simulink model "parte2_eje1_GeneradorSincrono"  (R2019b)
settings: Solver=VariableStepAuto  StartTime=0.0  StopTime=0.05  RelTol=1e-3
values from neighbouring files (symbols this model uses):
  id = It*sind(di+fi)    [parte2_eje1_GSin_constantes.m]
  ifd = (Et*cosd(di)+Ra*iq+Ld*id)/Lad    [parte2_eje1_GSin_constantes.m]
  iq = It*cosd(di+fi)    [parte2_eje1_GSin_constantes.m]
  L0 = 0.01    [parte2_eje1_GSin_constantes.m]
  L11d = 0.1713    [parte2_eje1_GSin_constantes.m]
  L11q = 0.7252    [parte2_eje1_GSin_constantes.m]
  L22q = 0.125    [parte2_eje1_GSin_constantes.m]
  Lad = sat*Lad    (= 1.38278)    [parte2_eje1_GSin_constantes.m]
  Laq = sat*Laq    (= 1.34113)    [parte2_eje1_GSin_constantes.m]
  Lf1d = 1.61    [parte2_eje1_GSin_constantes.m]
  Lffd = 0.165    [parte2_eje1_GSin_constantes.m]
  Ll = 0.15    [parte2_eje1_GSin_constantes.m]
  R1d = 0.0284    [parte2_eje1_GSin_constantes.m]
  R1q = 0.00619    [parte2_eje1_GSin_constantes.m]
  R2q = 0.02368    [parte2_eje1_GSin_constantes.m]
  Ra = 0.003    [parte2_eje1_GSin_constantes.m]
  Rfd = 0.0006    [parte2_eje1_GSin_constantes.m]
  th = 12*pi/180    (= 0.209439510239)    [parte2_eje1_GSin_constantes.m]
  wr = 1    [parte2_eje1_GSin_constantes.m]
settings Model: Creator=cjuar  LastModifiedBy=cjuar
settings DataIOCC: ReturnWorkspaceOutputs=off
settings DebuggingCC: ArithmeticOperatorsInVariantConditions=warning
settings SFSimCC: SimUseLocalCustomCode=off  CustomCodeUndefinedFunction=UseInterfaceOnly
settings RTWCC: RTWUseLocalCustomCode=off

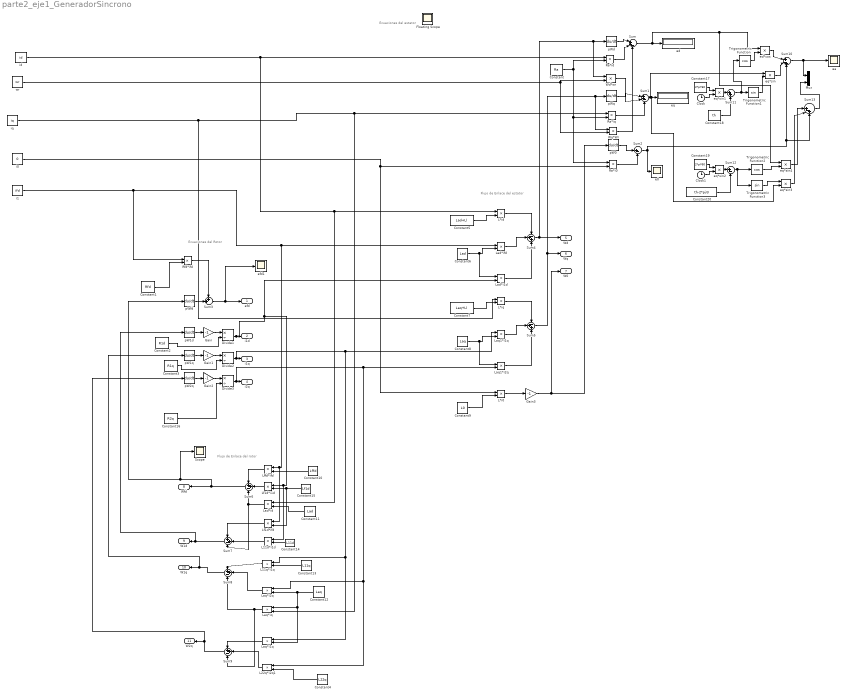
== system parte2_eje1_GeneradorSincrono ==
  note: Flujo de Enlace del estator
  note: Ecuaciones del Rotor
  note: Ecuaciones del estator
  note: Flujo de Enlace del rotor
  Clock : Clock
  Clock1 : Clock
  Constant : Constant  Value=Ra
  Constant1 : Constant  Value=Rfd
  Constant10 : Constant  Value=Lffd
  Constant11 : Constant  Value=Lad
  Constant12 : Constant  Value=Laq
  Constant13 : Constant  Value=L11q
  Constant14 : Constant  Value=L11d
  Constant15 : Constant  Value=Lf1d
  Constant16 : Constant  Value=R2q
  Constant17 : Constant  Value=2*pi*60
  Constant18 : Constant  Value=th
  Constant19 : Constant  Value=2*pi*60
  Constant2 : Constant  Value=R1d
  Constant20 : Constant  Value=th-2*pi/3
  Constant3 : Constant  Value=R1q
  Constant4 : Constant  Value=L22q
  Constant5 : Constant  Value=Lad+Ll
  Constant6 : Constant  Value=Lad
  Constant7 : Constant  Value=Laq+Ll
  Constant8 : Constant  Value=Laq
  Constant9 : Constant  Value=L0
  Divide1 : Product  Inputs=*/
  Divide2 : Product  Inputs=*/
  Divide3 : Product  Inputs=*/
  Floating Scope : Scope
      settings: Floating=on
  Gain{,1..3} (4 alike) : Gain  Gain=-1
  L*i0 : Product
  L*id : Product
  L*iq : Product
  L11d*i1d : Product
  L11q*i1q : Product
  L22q*i2q1 : Product
  Lad*i1d : Product
  Lad*id : Product
  Lad*ifd : Product
  Laq*i1q : Product
  Laq*i2q : Product
  Laq*iq : Product
  Laq1*i1q : Product
  Laq1*i2q : Product
  Lf1d*i1d : Product
  Lf1d*ifd : Product
  Lffd*ifd : Product
  Mux : Mux  Inputs=2
  Ra*i0 : Product
  Ra*id : Product
  "Ra*iq " : Product
  Rfd*ifd : Product
  Scope : Scope
  Sum : Sum  Inputs=|+--
  Sum1 : Sum  Inputs=|++-
  Sum10 : Sum  Inputs=|+-+
  Sum11 : Sum  Inputs=|++
  Sum12 : Sum  Inputs=|+-
  Sum13 : Sum  Inputs=||+-+
  Sum2 : Sum  Inputs=|+-
  Sum3 : Sum  Inputs=++|
  Sum4 : Sum  Inputs=-++
  Sum5 : Sum  Inputs=-++
  Sum{6..9} (4 alike) : Sum  Inputs=++-
  Trigonometric Function : Trigonometry  Operator=cos
  Trigonometric Function1 : Trigonometry
  Trigonometric Function2 : Trigonometry  Operator=cos
  Trigonometric Function3 : Trigonometry
  Wd*wr : Product
  Wq*Wr : Product
  e0 : Scope
  ea : Scope
  ed : Display
  ed*cos : Product
  efd1 : Scope
  eq : Display
  eq*sin{,1..4} (5 alike) : Product
  i0 : Constant  Value=0
  i1 : Constant  Value=ifd
  id : Constant  Value=id
  iq : Constant  Value=iq
  pW0 : Derivative
  pW1d : Derivative
  pW1q : Derivative
  pW2q : Derivative
  pWd : Derivative
  pWfd : Derivative
  pWq : Derivative
  wr : Constant  Value=wr
  efd : Outport  VectorParamsAs1DForOutWhenUnconnected=off
  i1d : Outport  Port=2  VectorParamsAs1DForOutWhenUnconnected=off
  i1q : Outport  Port=3  VectorParamsAs1DForOutWhenUnconnected=off
  i2q : Outport  Port=4  VectorParamsAs1DForOutWhenUnconnected=off
  Wd : Outport  Port=5  VectorParamsAs1DForOutWhenUnconnected=off
  Wq : Outport  Port=6  VectorParamsAs1DForOutWhenUnconnected=off
  W0 : Outport  Port=7  VectorParamsAs1DForOutWhenUnconnected=off
  Wfd : Outport  Port=8  VectorParamsAs1DForOutWhenUnconnected=off
  W1d : Outport  Port=9  VectorParamsAs1DForOutWhenUnconnected=off
  W1q : Outport  Port=10  VectorParamsAs1DForOutWhenUnconnected=off
  W2q : Outport  Port=11  VectorParamsAs1DForOutWhenUnconnected=off
  wires:
  Sum4/1 -> Wd/1, Wd*wr/1, pWd/1
  Sum5/1 -> Wq*Wr/1, pWq/1, Wq/1
  Gain3/1 -> W0/1, pW0/1
  wr/1 -> Wd*wr/2, Wq*Wr/2
  Sum/1 -> ed/1, eq*sin4/1, ed*cos/1
  pWd/1 -> Sum/1
  pWq/1 -> Sum1/1
  Sum1/1 -> eq*sin3/2, eq/1, eq*sin/1
  Wd*wr/1 -> Sum1/2
  Constant/1 -> Ra*id/2, Ra*i0/1, "Ra*iq "/2
  iq/1 -> "Ra*iq "/1, Laq*iq/2, L*iq/1
  Ra*id/1 -> Sum/2
  "Ra*iq "/1 -> Sum1/3
  i0/1 -> L*i0/1, Ra*i0/2
  Sum2/1 -> Sum13/3, Sum10/3, e0/1
  pW0/1 -> Sum2/1
  Ra*i0/1 -> Sum2/2
  Constant16/1 -> Divide3/2
  Constant3/1 -> Divide2/2
  Constant2/1 -> Divide1/2
  Constant1/1 -> Rfd*ifd/2
  Sum6/1 -> Scope/1, pWfd/1, Wfd/1
  Sum9/1 -> pW2q/1, W2q/1
  Sum8/1 -> pW1q/1, W1q/1
  Sum7/1 -> pW1d/1, W1d/1
  pWfd/1 -> Sum3/2
  i1/1 -> Rfd*ifd/1, Lad*ifd/1, Lf1d*ifd/1, Lffd*ifd/1
  pW1d/1 -> Gain/1
  Divide1/1 -> L11d*i1d/1, Lf1d*i1d/1, Lad*i1d/2, i1d/1
  Gain/1 -> Divide1/1
  pW1q/1 -> Gain1/1
  Gain1/1 -> Divide2/1
  Divide2/1 -> Laq*i1q/1, L11q*i1q/1, Laq1*i1q/1, i1q/1
  pW2q/1 -> Gain2/1
  Gain2/1 -> Divide3/1
  Divide3/1 -> Laq1*i2q/2, L22q*i2q1/1, Laq*i2q/1, i2q/1
  Wq*Wr/1 -> Sum/3
  Constant5/1 -> L*id/2
  L*id/1 -> Sum4/1
  Constant6/1 -> Lad*i1d/1, Lad*ifd/2
  Lad*i1d/1 -> Sum4/3
  Lad*ifd/1 -> Sum4/2
  Laq1*i1q/1 -> Sum5/2
  Laq1*i2q/1 -> Sum5/3
  Constant8/1 -> Laq1*i1q/2, Laq1*i2q/1
  L*iq/1 -> Sum5/1
  Constant7/1 -> L*iq/2
  Constant9/1 -> L*i0/2
  L*i0/1 -> Gain3/1
  Lf1d*i1d/1 -> Sum6/2
  Lad*id/1 -> Sum7/3, Sum6/3
  Lffd*ifd/1 -> Sum6/1
  Constant11/1 -> Lad*id/2
  id/1 -> L*id/1, Lad*id/1, Ra*id/1
  Constant15/1 -> Lf1d*ifd/2, Lf1d*i1d/2
  Constant14/1 -> L11d*i1d/2
  Constant13/1 -> L11q*i1q/2
  Constant10/1 -> Lffd*ifd/2
  Lf1d*ifd/1 -> Sum7/1
  L11d*i1d/1 -> Sum7/2
  Constant12/1 -> Laq*i1q/2, Laq*iq/1, Laq*i2q/2
  L11q*i1q/1 -> Sum8/1
  Laq*i2q/1 -> Sum8/2
  Laq*iq/1 -> Sum8/3, Sum9/3
  Laq*i1q/1 -> Sum9/1
  L22q*i2q1/1 -> Sum9/2
  Constant4/1 -> L22q*i2q1/2
  Rfd*ifd/1 -> Sum3/1
  Sum3/1 -> efd1/1, efd/1
  Trigonometric Function/1 -> ed*cos/2
  Trigonometric Function1/1 -> eq*sin/2
  eq*sin/1 -> Sum10/2
  ed*cos/1 -> Sum10/1
  Sum10/1 -> ea/1, Mux/1
  Constant17/1 -> eq*sin1/1
  Clock/1 -> eq*sin1/2
  eq*sin1/1 -> Sum11/1
  Sum11/1 -> Trigonometric Function/1, Trigonometric Function1/1
  Constant18/1 -> Sum11/2
  Constant20/1 -> Sum12/2
  eq*sin2/1 -> Sum12/1
  Clock1/1 -> eq*sin2/2
  Constant19/1 -> eq*sin2/1
  Sum12/1 -> Trigonometric Function3/1, Trigonometric Function2/1
  Trigonometric Function2/1 -> eq*sin4/2
  Trigonometric Function3/1 -> eq*sin3/1
  eq*sin4/1 -> Sum13/1
  eq*sin3/1 -> Sum13/2
  Sum13/1 -> Mux/2
